simulink model "TwoTank"  (R2016a)
settings: Solver=ode45  StartTime=0.0  StopTime=inputOpt.simTime  RelTol=1e-3
undefined symbols (not defined in the file): Initials, inputOpt, L1i, L2i, T1i, T2i
libraries: TTLibrary x12
settings Model: Creator=blindner  LastModifiedBy=blindner
settings DataIOCC: SaveFormat=Array  InspectSignalLogs=on
settings HardwareCC: ProdBitPerPointer=32  ProdLargestAtomicFloat=None  ProdIntDivRoundTo=Undefined  ProdEndianess=Unspecified  ProdWordSize=32  ProdHWDeviceType=32-bit Generic
settings ModelReferenceCC: PropagateSignalLabelsOutOfModel=off
settings ConfigComp: CovModelRefEnable=Off

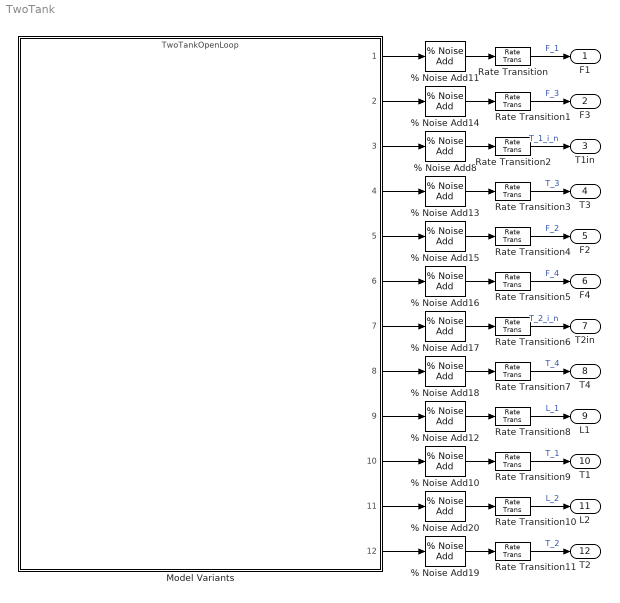
== system TwoTank ==
  % Noise Add10 : TTLibrary/% Noise Add  perc=percN  seed=randi(100000)  addNoiseMult=1  Ts=inputOpt.sampleTime  noiseAmp=T1i
  % Noise Add11 : TTLibrary/% Noise Add  perc=percN  seed=randi(100000)  addNoiseMult=inputOpt.addNoise  Ts=inputOpt.sampleTime  noiseAmp=Initials.F1
  % Noise Add12 : TTLibrary/% Noise Add  perc=percN  seed=randi(100000)  addNoiseMult=inputOpt.addNoise  Ts=inputOpt.sampleTime  noiseAmp=L1i
  % Noise Add13 : TTLibrary/% Noise Add  perc=percN  seed=randi(100000)  addNoiseMult=inputOpt.addNoise  Ts=inputOpt.sampleTime  noiseAmp=inputOpt.T3.start
  % Noise Add14 : TTLibrary/% Noise Add  perc=percN  seed=randi(100000)  addNoiseMult=inputOpt.addNoise  Ts=inputOpt.sampleTime  noiseAmp=Initials.F3
  % Noise Add15 : TTLibrary/% Noise Add  perc=percN  seed=randi(100000)  addNoiseMult=inputOpt.addNoise  Ts=inputOpt.sampleTime  noiseAmp=Initials.F2
  % Noise Add16 : TTLibrary/% Noise Add  perc=percN  seed=randi(100000)  addNoiseMult=inputOpt.addNoise  Ts=inputOpt.sampleTime  noiseAmp=Initials.F4
  % Noise Add17 : TTLibrary/% Noise Add  perc=percN  seed=randi(100000)  addNoiseMult=inputOpt.addNoise  Ts=inputOpt.sampleTime  noiseAmp=inputOpt.T2in.start
  % Noise Add18 : TTLibrary/% Noise Add  perc=percN  seed=randi(100000)  addNoiseMult=inputOpt.addNoise  Ts=inputOpt.sampleTime  noiseAmp=inputOpt.T4.start
  % Noise Add19 : TTLibrary/% Noise Add  perc=percN  seed=randi(100000)  addNoiseMult=inputOpt.addNoise  Ts=inputOpt.sampleTime  noiseAmp=T2i
  % Noise Add20 : TTLibrary/% Noise Add  perc=percN  seed=randi(100000)  addNoiseMult=inputOpt.addNoise  Ts=inputOpt.sampleTime  noiseAmp=L2i
  % Noise Add8 : TTLibrary/% Noise Add  perc=percN  seed=randi(100000)  addNoiseMult=inputOpt.addNoise  Ts=inputOpt.sampleTime  noiseAmp=inputOpt.T1in.start
  Model Variants : ModelReference  ModelNameDialog=TwoTankOpenLoop.slx  SimulationMode=Normal  Variant=on  ModelReferenceVersion=1.263
      settings: AttributesFormatString=%<ActiveVariant>
  Rate Transition : RateTransition  X0=Initials.F1  OutPortSampleTime=inputOpt.sampleTime
  Rate Transition1 : RateTransition  X0=Initials.F3  OutPortSampleTime=inputOpt.sampleTime
  Rate Transition10 : RateTransition  X0=L2i  OutPortSampleTime=inputOpt.sampleTime
  Rate Transition11 : RateTransition  X0=T2i  OutPortSampleTime=inputOpt.sampleTime
  Rate Transition2 : RateTransition  X0=inputOpt.T1in.start  OutPortSampleTime=inputOpt.sampleTime
  Rate Transition3 : RateTransition  X0=inputOpt.T3.start  OutPortSampleTime=inputOpt.sampleTime
  Rate Transition4 : RateTransition  X0=Initials.F2  OutPortSampleTime=inputOpt.sampleTime
  Rate Transition5 : RateTransition  X0=Initials.F4  OutPortSampleTime=inputOpt.sampleTime
  Rate Transition6 : RateTransition  X0=inputOpt.T2in.start  OutPortSampleTime=inputOpt.sampleTime
  Rate Transition7 : RateTransition  X0=inputOpt.T4.start  OutPortSampleTime=inputOpt.sampleTime
  Rate Transition8 : RateTransition  X0=L1i  OutPortSampleTime=inputOpt.sampleTime
  Rate Transition9 : RateTransition  X0=T1i  OutPortSampleTime=inputOpt.sampleTime
  F1 : Outport  SampleTime=inputOpt.sampleTime
  F3 : Outport  Port=2  SampleTime=inputOpt.sampleTime
  T1in : Outport  Port=3  SampleTime=inputOpt.sampleTime
  T3 : Outport  Port=4  SampleTime=inputOpt.sampleTime
  F2 : Outport  Port=5  SampleTime=inputOpt.sampleTime
  F4 : Outport  Port=6  SampleTime=inputOpt.sampleTime
  T2in : Outport  Port=7  SampleTime=inputOpt.sampleTime
  T4 : Outport  Port=8  SampleTime=inputOpt.sampleTime
  L1 : Outport  Port=9  OutDataTypeStr=double  PortDimensions=1  SampleTime=inputOpt.sampleTime
  T1 : Outport  Port=10  OutDataTypeStr=double  PortDimensions=1  SampleTime=inputOpt.sampleTime
  L2 : Outport  Port=11  OutDataTypeStr=double  PortDimensions=1  SampleTime=inputOpt.sampleTime
  T2 : Outport  Port=12  OutDataTypeStr=double  PortDimensions=1  SampleTime=inputOpt.sampleTime
  wires:
  Model Variants/10 -> % Noise Add10/1
  Model Variants/1 -> % Noise Add11/1
  Model Variants/4 -> % Noise Add13/1
  Model Variants/3 -> % Noise Add8/1
  Model Variants/2 -> % Noise Add14/1
  Model Variants/6 -> % Noise Add16/1
  Model Variants/5 -> % Noise Add15/1
  Model Variants/9 -> % Noise Add12/1
  Model Variants/8 -> % Noise Add18/1
  Model Variants/7 -> % Noise Add17/1
  Model Variants/11 -> % Noise Add20/1
  Model Variants/12 -> % Noise Add19/1
  Rate Transition/1 -> F1/1  "F_1"
  Rate Transition1/1 -> F3/1  "F_3"
  Rate Transition2/1 -> T1in/1  "T_1_i_n"
  Rate Transition3/1 -> T3/1  "T_3"
  Rate Transition4/1 -> F2/1  "F_2"
  Rate Transition5/1 -> F4/1  "F_4"
  Rate Transition6/1 -> T2in/1  "T_2_i_n"
  Rate Transition7/1 -> T4/1  "T_4"
  Rate Transition8/1 -> L1/1  "L_1"
  Rate Transition9/1 -> T1/1  "T_1"
  Rate Transition10/1 -> L2/1  "L_2"
  Rate Transition11/1 -> T2/1  "T_2"
  % Noise Add11/1 -> Rate Transition/1
  % Noise Add14/1 -> Rate Transition1/1
  % Noise Add8/1 -> Rate Transition2/1
  % Noise Add13/1 -> Rate Transition3/1
  % Noise Add15/1 -> Rate Transition4/1
  % Noise Add16/1 -> Rate Transition5/1
  % Noise Add17/1 -> Rate Transition6/1
  % Noise Add18/1 -> Rate Transition7/1
  % Noise Add12/1 -> Rate Transition8/1
  % Noise Add10/1 -> Rate Transition9/1
  % Noise Add20/1 -> Rate Transition10/1
  % Noise Add19/1 -> Rate Transition11/1
